simulink model "Function6_2018a"  (R2018a)
settings: Solver=FixedStepDiscrete  StartTime=0.0  StopTime=0.1  FixedStep=0.1  RelTol=1e-3  EnableMultiTasking=on
settings Model: Creator=bzhan  LastModifiedBy=bzhan
settings SolverCC: AutoInsertRateTranBlk=on
settings DataIOCC: LimitDataPoints=on  ReturnWorkspaceOutputs=on
settings OptimizationCC: LifeSpan=inf
settings DebuggingCC: AllowSymbolicDim=off  SFUnexpectedBacktrackingDiag=warning  SFNoUnconditionalDefaultTransitionDiag=warning  SFExecutionAtInitializationDiag=none
settings CodeAppCC: StateflowObjectComments=on
settings GRTTargetCC: TargetLangStandard=C89/C90 (ANSI)
settings ConfigComp: CovMetricSettings=dw  CovHtmlReporting=on  CovSaveCumulativeToWorkspaceVar=on  CovSaveSingleToWorkspaceVar=on  CovShowResultsExplorer=off  CovExternalEMLEnable=off  CovSFcnEnable=off

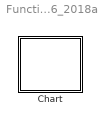
== system Function6_2018a ==
  Chart : Stateflow chart  TreatAsAtomicUnit=on

== stateflow chart Function6_2018a/Chart ==
  state A
    en: f("en_A")
  state B
    en: f("en_B")
  (default) -> A : {b=[0 1 2 3];}
  A -> (junction 29) : {compute()}
  (junction 29) -> B : [a(3)==2 && b(3)==3]
  data: s function_input; b local double size=1 4 =[0 0 0 0]; a local size=1 4 =[0 0 0 0]
  function compute:
    | function compute
    |   a = b;
    |   b(3) = 3;
  function f(s):
    | function f(s)
    |   fprintf(s+"\n");
